simulink model "model_FedBatch"  (R2025b)
settings: Solver=VariableStepAuto  StartTime=0.0  StopTime=36000  RelTol=1e-3
libraries: ChemReactorDesign_lib x8, nesl_utility x3
settings Model: Creator=klaus  LastModifiedBy=klaus
settings SolverCC: ZeroCrossAlgorithm=Adaptive
settings DebuggingCC: IgnoredZcDiagnostic=none
settings RTWCC: GPUComputeCapability=3.5
settings SimscapeCC: SimscapeLogType=all

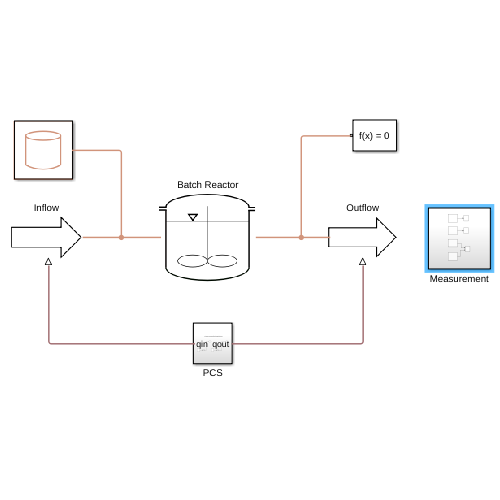
[thumbnail: Simulink's stored preview of the top-level diagram]
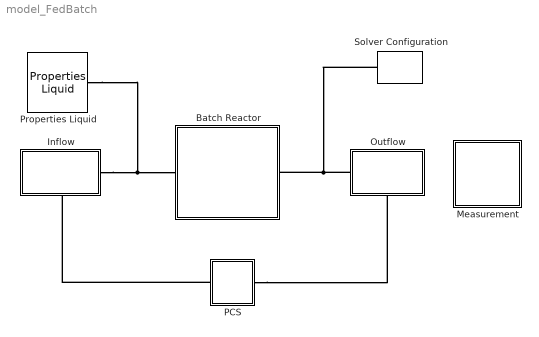
== system model_FedBatch ==
  Batch Reactor : Subsystem
  Inflow : Subsystem
      settings: PortSchema="{\"entries\":[{\"content\":{\"sides\":[{\"content\":{},\"type\":\"ConnectorPlacement.EquallySpacedRectSide\",\"uuid\":\"dd183d82-0f77-49b2-92e8-991cd411421b\"},{\"content\":{\"connectorIds\":[\"RConn1\"],\"side\":\"RIGHT\"},\"type\":\"ConnectorPlacement.EquallySpacedRectSide\",\"uuid\":\"300d84b6-2169-47ab-91d0-57398ce60882\"},{\"content\":{\"side\":\"TOP\"},\"type\":\"ConnectorPlacement.EquallySpacedRectSide\",\"uuid\":\"f69a5909-efdd-48cc-a251-60512357e348\"},{\"content\":{\"connectorIds\":[\"RConn2\"],\"side\":\"BOTTOM\"},\"type\":\"ConnectorPlacement.EquallySpacedRectSide\",\"uuid\":\"6d14b4c2-5fd4-4caf-b374-e5929d10ca28\"}]},\"type\":\"ConnectorPlacement.EquallySpacedConnector\",\"uuid\":\"c1864954-4e61-47a7-87b5-5378b3d024af\"}],\"packageUris\":[\"http://schema.mathworks.com/mf0/Connector/R2020b\"],\"version\":\"1.0\"}"
  Measurement : Subsystem
  Outflow : Subsystem
      settings: PortSchema="{\"entries\":[{\"content\":{\"sides\":[{\"content\":{\"connectorIds\":[\"LConn1\"]},\"type\":\"ConnectorPlacement.EquallySpacedRectSide\",\"uuid\":\"43eb4d57-857c-42ed-87a1-67f97bf0db74\"},{\"content\":{\"side\":\"RIGHT\"},\"type\":\"ConnectorPlacement.EquallySpacedRectSide\",\"uuid\":\"a8e30eb6-f3c3-4987-82b8-87f74520922e\"},{\"content\":{\"side\":\"TOP\"},\"type\":\"ConnectorPlacement.EquallySpacedRectSide\",\"uuid\":\"fcc232a9-b129-407f-9ca1-711f21c5b310\"},{\"content\":{\"connectorIds\":[\"RConn1\"],\"side\":\"BOTTOM\"},\"type\":\"ConnectorPlacement.EquallySpacedRectSide\",\"uuid\":\"8236142f-b7ec-4603-bf4f-23f510a75819\"}]},\"type\":\"ConnectorPlacement.EquallySpacedConnector\",\"uuid\":\"e9c3614e-93bb-4134-9328-a8e1dc61e4da\"}],\"packageUris\":[\"http://schema.mathworks.com/mf0/Connector/R2020b\"],\"version\":\"1.0\"}"
  PCS : Subsystem
  Properties Liquid : ChemReactorDesign_lib/Basic/Liquid/Utilities/Properties Liquid  model=ChemReactorDesign.Basic.Liquid.enum.ThermodynamicModel.Ideal  N=3  Ids=[12;13;1]  Mw=[0;0;18.0153] g/mol  charge=[0;0;0]  table_T=[290 300] K  table_cp=[0 0 75.5402184579739;0 0 75.5425835956457] J/(K*mol)  table_Vm=[0 0 0.0180471322987256;0 0 0.018091238618091] l/mol  table_H=[0 0 -286.738719251556;0 0 -285.574694009364] kJ/mol  table_G=[0 0 -241.603407405;0 0 -239.651281374905] kJ/mol  table_mu=[0 0 0.00109430979865936;0 0 0.000860172426313474] Pa*s  table_lambda=[0 0 0.597518852340043;0 0 0.612989139138324] W/(K*m)  table_Hv=[0 0 44.3090602722826;0 0 43.9004472013488] kJ/mol  table_pvap=[0 0 1921.03049696876;0 0 3541.05430536848] Pa  A=[1 0 0;0 1 0;0 0 1] cal/mol  alpha=[0 0 0;0 0 0;0 0 0]  F_nom=1.0e-06 mol/s  Phi_nom=1.0 W  Q_nom=1.0 W  H_nom=1.0e+02 kJ/mol
      settings: SourceProductName=Chemical Reactor Design ToolBox  InternalSimscapePortConfiguration="{\"Bottom\":[],\"Left\":[],\"Right\":[{\"id\":\"Port_B\",\"label\":\"\",\"type\":\"ChemReactorDesign.Basic.Liquid.Liquid\"}],\"Top\":[]}"
  Solver Configuration : nesl_utility/Solver Configuration  PhysicalDomain=network_engine_domain  SubClassName=solver  LeftPortType=input  RightPortType=generic  Tones=[]  Harmonics=[]  SimulateNoise=off  Profile=off  UseLocalSampling=off  EnableSwitchedLinearOptims=on  FrequencyDomain=off  UseCCode=off  RelTol=0.001  AbsTol=0.001  MinStep=1e-09  ToWorkspace=off  RevertToSquareIcSolve=off  NumHomotopyIterations=100  PhasorMode=off  PhasorModeNumHarmonics=1  ConsistencySolver=NEWTON_XTOL_AFTER_FTOL  IndexReductionMethod=DerivativeReplacement  DoDC=off  ResidualTolerance=1e-09  ConsistencyTolSource=GLOBAL  ConsistencyAbsTol=0.001  ConsistencyRelTol=0.001  ConsistencyTolFactor=0.001  UseLocalSolver=off  LocalSolverChoice=NE_BACKWARD_EULER_ADVANCER  ResolveIndetEquations=on  FunctionEvalNumThread=1  LocalSolverSampleTime=0.001  DoFixedCost=off  MaxNonlinIter=3  MaxModeIter=2  ComputeImpulses=off  ImpulseIterations=2  LinearAlgebra=auto  LinearAlgebraNumThread=0  EquationFormulation=NE_TIME_EF  DelaysMemoryBudget=1024  AutomaticFiltering=on  FilteringTimeConstant=0.001  PartitionStorageMethod=AS_NEEDED  PartitionMemoryBudget=1024  PartitionMethod=ROBUST  MultibodyUseLocalSolver=off  MultibodyLocalSolverChoice=ODE1  MultibodyLocalSolverSampleTime=0.001
  connections:
  Outflow/LConn1 -- Solver Configuration/RConn1 -- Batch Reactor/RConn1
  PCS/LConn1 -- Inflow/RConn2
  PCS/RConn1 -- Outflow/RConn1
  Properties Liquid/RConn1 -- Inflow/RConn1 -- Batch Reactor/LConn1

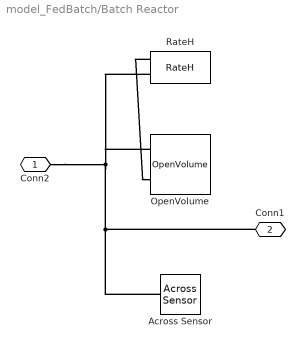
== system model_FedBatch/Batch Reactor ==
  Across Sensor : ChemReactorDesign_lib/Basic/Liquid/Sensors/Across Sensor  concentrationsOutput=ChemReactorDesign.Basic.enum.OnOff.On  temperatureOutput=ChemReactorDesign.Basic.enum.OnOff.Off  pressureOutput=ChemReactorDesign.Basic.enum.OnOff.Off  fractionsOutput=ChemReactorDesign.Basic.enum.OnOff.Off  selectSpecies=[1, 2]
      settings: SourceProductName=Chemical Reactor Design ToolBox  InternalSimscapePortConfiguration="{\"Bottom\":[],\"Left\":[{\"id\":\"Port_A\",\"label\":\"\",\"type\":\"ChemReactorDesign.Basic.Liquid.Liquid\"}],\"Right\":[{\"id\":\"cout\",\"label\":\"c\",\"type\":\"output\"}],\"Top\":[]}"
  OpenVolume : ChemReactorDesign_lib/Basic/Liquid/Volumes/OpenVolume  pressureInput=ChemReactorDesign.Basic.enum.OnOff.Off  volumeOutput=ChemReactorDesign.Basic.enum.OnOff.On  isothermalOperation=ChemReactorDesign.Basic.enum.OnOff.On  V0=0.1 m^3  A0=1 m^2  h0=0 m  x0=[0.0350262697022767 0.00175131348511384 0.963222416812609]  p0=1 bar  T0=298.15 K  n_nom=1 mol
      settings: SourceProductName=Chemical Reactor Design ToolBox  InternalSimscapePortConfiguration="{\"Bottom\":[],\"Left\":[{\"id\":\"Port_A\",\"label\":\"\",\"type\":\"ChemReactorDesign.Basic.Liquid.Liquid\"}],\"Right\":[],\"Top\":[{\"id\":\"Vout\",\"label\":\"V\",\"type\":\"output\"}]}"
  RateH : ChemReactorDesign_lib/Basic/Liquid/Rates/RateH  rateReference=ChemReactorDesign.Basic.enum.RateReference.Volume  reversibility=ChemReactorDesign.Basic.enum.Reversibility.Irreversible  nu=[-1;1;0]  calculate_Ka=ChemReactorDesign.Basic.enum.OnOff.Off  Ka0=1.0e+30  kfinfV=0.8 mol/(hr*l)  kfinfA=0 mol/(cm^2*s)  kfinfm=0 mol/(g*s)  Ea=0 kJ/mol  kappaf=[1;1;0]  beta0=0.1  betainf=1  Es=0 kJ/mol  kappak=[1;0;0]  n=1
      settings: SourceProductName=Chemical Reactor Design ToolBox  InternalSimscapePortConfiguration="{\"Bottom\":[],\"Left\":[{\"id\":\"Port_B\",\"label\":\"\",\"type\":\"ChemReactorDesign.Basic.Liquid.Liquid\"}],\"Right\":[],\"Top\":[{\"id\":\"V\",\"label\":\"V\",\"type\":\"input\"}]}"
  Conn2 : PMIOPort  Side=Left
  Conn1 : PMIOPort  Port=2  Side=Right
  connections:
  Conn2/RConn1 -- Conn1/RConn1 -- Across Sensor/LConn1 -- RateH/LConn1 -- OpenVolume/LConn1
  RateH/LConn2 -- OpenVolume/LConn2

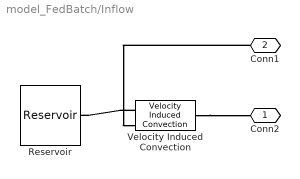
== system model_FedBatch/Inflow ==
  Reservoir : ChemReactorDesign_lib/Basic/Liquid/Utilities/Reservoir  x0=[0.0833333333333333 0 0.916666666666667]  p0=1 bar  T0=298.15 K
      settings: SourceProductName=Chemical Reactor Design ToolBox  InternalSimscapePortConfiguration="{\"Bottom\":[],\"Left\":[{\"id\":\"Port_A\",\"label\":\"\",\"type\":\"ChemReactorDesign.Basic.Liquid.Liquid\"}],\"Right\":[],\"Top\":[]}"
  Velocity Induced Convection : ChemReactorDesign_lib/Basic/Liquid/Transport/Velocity Induced Convection  flowInput=ChemReactorDesign.Basic.enum.OnOff.On  controlInput=ChemReactorDesign.Basic.enum.OnOff.Off  q0=0.1 m^3/hr  areaInput=ChemReactorDesign.Basic.enum.OnOff.Off  A0=1 m^2  delta=1.0e-03 m  flowOutput=ChemReactorDesign.Basic.enum.OnOff.Off  checkValve=ChemReactorDesign.Basic.enum.OnOff.Off  ymin=1.0e-10  q_specify=off  q_priority=None  q=0 l/s  q_nominal_specify=off  q_nominal_value=1  q_nominal_unit=l/s
      settings: SourceProductName=Chemical Reactor Design ToolBox  InternalSimscapePortConfiguration="{\"Bottom\":[],\"Left\":[{\"id\":\"Port_A\",\"label\":\"\",\"type\":\"ChemReactorDesign.Basic.Liquid.Liquid\"}],\"Right\":[{\"id\":\"Port_B\",\"label\":\"\",\"type\":\"ChemReactorDesign.Basic.Liquid.Liquid\"}],\"Top\":[{\"id\":\"qin\",\"label\":\"q\",\"type\":\"input\"}]}"
  Conn2 : PMIOPort  Side=Right
  Conn1 : PMIOPort  Port=2  Side=Right
  connections:
  Velocity Induced Convection/RConn1 -- Conn2/RConn1
  Velocity Induced Convection/LConn1 -- Reservoir/LConn1
  Conn1/RConn1 -- Velocity Induced Convection/LConn2

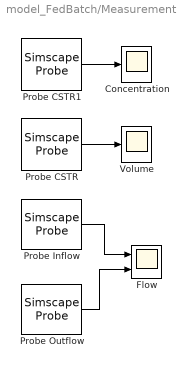
== system model_FedBatch/Measurement ==
  Concentration : Scope
      settings: ActiveDisplayYMinimum=-0.5879149873370848  ActiveDisplayYMaximum=5.2912348860337639  DataLoggingVariableName=ScopeData2
  Flow : Scope  NumInputPorts=2
      settings: ActiveDisplayYMinimum=-0.013888888888888886  ActiveDisplayYMaximum=0.125
  Probe CSTR : SimscapeProbe  BoundBlock=114  Variables="{\"V\":{\"Probing\":\"ON\"},\"Vout\":{\"Probing\":\"OFF\"}}"
  Probe CSTR1 : SimscapeProbe  BoundBlock=115  Variables="{\"cout\":{\"Probing\":\"ON\"}}"
  Probe Inflow : SimscapeProbe  BoundBlock=110  Variables="{\"qin\":{\"Probing\":\"ON\"}}"
  Probe Outflow : SimscapeProbe  BoundBlock=111  Variables="{\"qin\":{\"Probing\":\"ON\"}}"
  Volume : Scope
      settings: ActiveDisplayYMinimum=-1.6792123247455493E-15  ActiveDisplayYMaximum=1.0000000000000027  DataLoggingVariableName=ScopeData3
  wires:
  Probe Outflow/1 -> Flow/2
  Probe Inflow/1 -> Flow/1
  Probe CSTR/1 -> Volume/1
  Probe CSTR1/1 -> Concentration/1

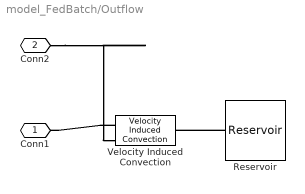
== system model_FedBatch/Outflow ==
  Reservoir : ChemReactorDesign_lib/Basic/Liquid/Utilities/Reservoir  x0=[0;0;1]  p0=1 bar  T0=298.15 K
      settings: SourceProductName=Chemical Reactor Design ToolBox  InternalSimscapePortConfiguration="{\"Bottom\":[],\"Left\":[{\"id\":\"Port_A\",\"label\":\"\",\"type\":\"ChemReactorDesign.Basic.Liquid.Liquid\"}],\"Right\":[],\"Top\":[]}"
  Velocity Induced Convection : ChemReactorDesign_lib/Basic/Liquid/Transport/Velocity Induced Convection  flowInput=ChemReactorDesign.Basic.enum.OnOff.On  controlInput=ChemReactorDesign.Basic.enum.OnOff.Off  q0=0 l/min  areaInput=ChemReactorDesign.Basic.enum.OnOff.Off  A0=1 m^2  delta=1.0e-03 m  flowOutput=ChemReactorDesign.Basic.enum.OnOff.Off  checkValve=ChemReactorDesign.Basic.enum.OnOff.Off  ymin=1.0e-10  q_specify=off  q_priority=None  q=0 l/s  q_nominal_specify=off  q_nominal_value=1  q_nominal_unit=l/s
      settings: SourceProductName=Chemical Reactor Design ToolBox  InternalSimscapePortConfiguration="{\"Bottom\":[],\"Left\":[{\"id\":\"Port_A\",\"label\":\"\",\"type\":\"ChemReactorDesign.Basic.Liquid.Liquid\"}],\"Right\":[{\"id\":\"Port_B\",\"label\":\"\",\"type\":\"ChemReactorDesign.Basic.Liquid.Liquid\"}],\"Top\":[{\"id\":\"qin\",\"label\":\"q\",\"type\":\"input\"}]}"
  Conn1 : PMIOPort  Side=Left
  Conn2 : PMIOPort  Port=2  Side=Right
  connections:
  Conn2/RConn1 -- Velocity Induced Convection/LConn2
  Reservoir/LConn1 -- Velocity Induced Convection/RConn1
  Velocity Induced Convection/LConn1 -- Conn1/RConn1

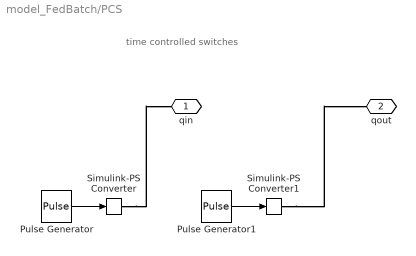
== system model_FedBatch/PCS ==
  note: time controlled switches
  Pulse Generator : DiscretePulseGenerator  PulseType=Time based  Amplitude=0.1  Period=36000  PulseWidth=80
  Pulse Generator1 : DiscretePulseGenerator  PulseType=Time based  Amplitude=0.4  Period=36000  PulseWidth=20  PhaseDelay=28800
  Simulink-PS Converter : nesl_utility/Simulink-PS Converter  PhysicalDomain=network_engine_domain  SubClassName=ps_input  LeftPortType=input  RightPortType=output  PseudoPeriodic=off  Frequencies=[]  NoiseDistribution=none  NoiseParameters=[]  Unit=m^3/hr  AffineConversion=off  FilteringAndDerivatives=provide  SimscapeFilterOrder=1  InputFilterTimeConstant=0.001  UdotUserProvided=0
  Simulink-PS Converter1 : nesl_utility/Simulink-PS Converter  PhysicalDomain=network_engine_domain  SubClassName=ps_input  LeftPortType=input  RightPortType=output  PseudoPeriodic=off  Frequencies=[]  NoiseDistribution=none  NoiseParameters=[]  Unit=m^3/hr  AffineConversion=off  FilteringAndDerivatives=provide  SimscapeFilterOrder=1  InputFilterTimeConstant=0.001  UdotUserProvided=0
  qin : PMIOPort  Side=Left
  qout : PMIOPort  Port=2  Side=Right
  wires:
  Pulse Generator/1 -> Simulink-PS Converter/1
  Pulse Generator1/1 -> Simulink-PS Converter1/1
  connections:
  Simulink-PS Converter/RConn1 -- qin/RConn1
  Simulink-PS Converter1/RConn1 -- qout/RConn1
